simulink model "SimplePendulumControl"  (R2025b)
settings: Solver=VariableStepAuto  StartTime=0.0  StopTime=10  RelTol=1e-3
settings Model: Creator=alvaro  LastModifiedBy=alvaro

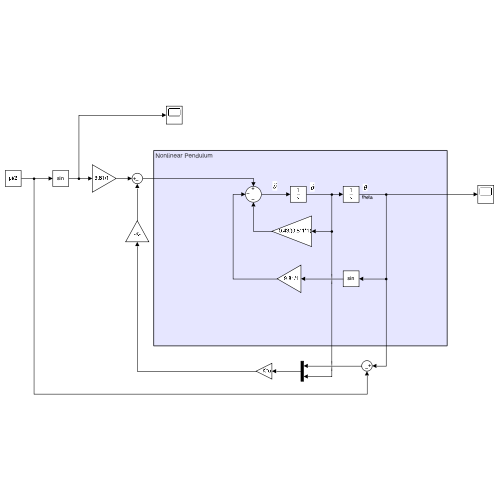
[thumbnail: Simulink's stored preview of the top-level diagram]
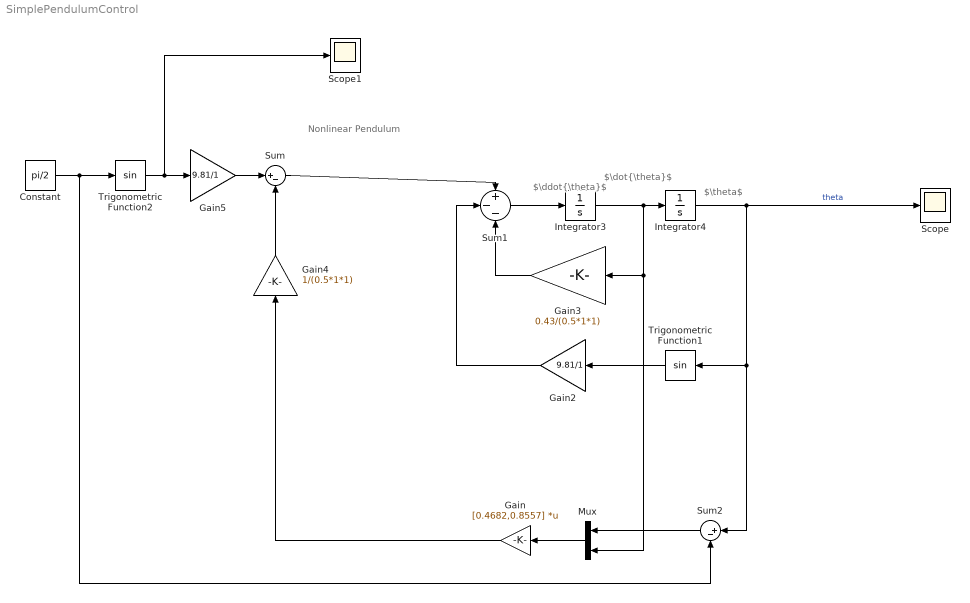
== system SimplePendulumControl ==
  note: $\theta$
  note: Nonlinear Pendulum
  note: $\dot{\theta}$
  note: $\ddot{\theta}$
  Constant : Constant  Value=pi/2  SampleTime=-1
  Gain : Gain  Gain=[0.4682,0.8557]  Multiplication=Matrix(K*u)
  Gain2 : Gain  Gain=9.81/1
  Gain3 : Gain  Gain=0.43/(0.5*1*1)
  Gain4 : Gain  Gain=1/(0.5*1*1)
  Gain5 : Gain  Gain=9.81/1
  Integrator3 : Integrator
  Integrator4 : Integrator  InitialCondition=pi/2 - 0.1
  Mux : Mux  Inputs=2
  Scope : Scope
      settings: ActiveDisplayYMinimum=1.4584007046693928  ActiveDisplayYMaximum=1.5823569259244303
  Scope1 : Scope
      settings: ActiveDisplayYMinimum=0.9  ActiveDisplayYMaximum=1.1
  Sum : Sum  Inputs=|+-
  Sum1 : Sum  Inputs=+--
  Sum2 : Sum  Inputs=|+-
  Trigonometric Function1 : Trigonometry
  Trigonometric Function2 : Trigonometry
  wires:
  Sum1/1 -> Integrator3/1
  Integrator3/1 -> Mux/2, Gain3/1, Integrator4/1
  Integrator4/1 -> Sum2/1, Trigonometric Function1/1, Scope/1  "theta"
  Trigonometric Function1/1 -> Gain2/1
  Constant/1 -> Sum2/2, Trigonometric Function2/1
  Trigonometric Function2/1 -> Scope1/1, Gain5/1
  Mux/1 -> Gain/1
  Gain3/1 -> Sum1/3
  Gain2/1 -> Sum1/2
  Gain/1 -> Gain4/1
  Sum2/1 -> Mux/1
  Gain5/1 -> Sum/1
  Sum/1 -> Sum1/1
  Gain4/1 -> Sum/2
